simulink model "unitdelay_test"  (Simulink 7.2)
settings: Solver=ode45  StartTime=0.0  StopTime=10.0  RelTol=1e-3
settings Model: Creator=arnaud  LastModifiedBy=arnaud
settings DataIOCC: SaveFormat=Structure

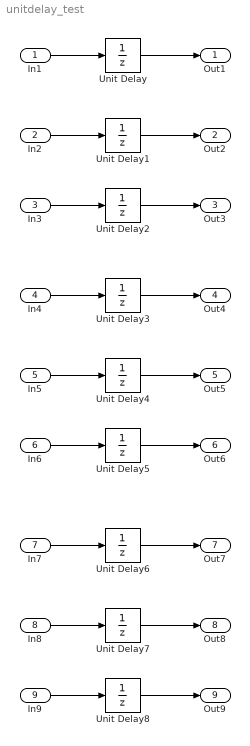
== system unitdelay_test ==
  In1 : Inport  PortDimensions=1  DataType=double  OutDataType=sfix(16)  OutScaling=2^0  OutDataTypeStr=double
  In2 : Inport  Port=2  PortDimensions=1  DataType=double  OutDataType=sfix(16)  OutScaling=2^0  OutDataTypeStr=double
  In3 : Inport  Port=3  PortDimensions=1  OutDataType=sfix(16)  OutScaling=2^0
  In4 : Inport  Port=4  PortDimensions=1  DataType=int8  OutDataType=sfix(16)  OutScaling=2^0  OutDataTypeStr=int8
  In5 : Inport  Port=5  PortDimensions=1  DataType=int8  OutDataType=sfix(16)  OutScaling=2^0  OutDataTypeStr=int8
  In6 : Inport  Port=6  PortDimensions=1  DataType=int8  OutDataType=sfix(16)  OutScaling=2^0  OutDataTypeStr=int8
  In7 : Inport  Port=7  PortDimensions=1  DataType=boolean  OutDataType=sfix(16)  OutScaling=2^0  OutDataTypeStr=boolean
  In8 : Inport  Port=8  PortDimensions=1  DataType=boolean  OutDataType=sfix(16)  OutScaling=2^0  OutDataTypeStr=boolean
  In9 : Inport  Port=9  PortDimensions=1  DataType=boolean  OutDataType=sfix(16)  OutScaling=2^0  OutDataTypeStr=boolean
  Unit Delay : UnitDelay
  Unit Delay1 : UnitDelay  X0=0.0
  Unit Delay2 : UnitDelay  X0=true
  Unit Delay3 : UnitDelay
  Unit Delay4 : UnitDelay  X0=0.0
  Unit Delay5 : UnitDelay  X0=true
  Unit Delay6 : UnitDelay
  Unit Delay7 : UnitDelay  X0=0.0
  Unit Delay8 : UnitDelay  X0=true
  Out1 : Outport  OutDataType=sfix(16)  OutScaling=2^0
  Out2 : Outport  Port=2  OutDataType=sfix(16)  OutScaling=2^0
  Out3 : Outport  Port=3  OutDataType=sfix(16)  OutScaling=2^0
  Out4 : Outport  Port=4  OutDataType=sfix(16)  OutScaling=2^0
  Out5 : Outport  Port=5  OutDataType=sfix(16)  OutScaling=2^0
  Out6 : Outport  Port=6  OutDataType=sfix(16)  OutScaling=2^0
  Out7 : Outport  Port=7  OutDataType=sfix(16)  OutScaling=2^0
  Out8 : Outport  Port=8  OutDataType=sfix(16)  OutScaling=2^0
  Out9 : Outport  Port=9  OutDataType=sfix(16)  OutScaling=2^0
  wires:
  In1/1 -> Unit Delay/1
  Unit Delay/1 -> Out1/1
  In2/1 -> Unit Delay1/1
  Unit Delay1/1 -> Out2/1
  In3/1 -> Unit Delay2/1
  Unit Delay2/1 -> Out3/1
  In4/1 -> Unit Delay3/1
  Unit Delay3/1 -> Out4/1
  In5/1 -> Unit Delay4/1
  Unit Delay4/1 -> Out5/1
  In6/1 -> Unit Delay5/1
  Unit Delay5/1 -> Out6/1
  In7/1 -> Unit Delay6/1
  Unit Delay6/1 -> Out7/1
  In8/1 -> Unit Delay7/1
  Unit Delay7/1 -> Out8/1
  In9/1 -> Unit Delay8/1
  Unit Delay8/1 -> Out9/1
